simulink model "tempReflexBlockBKP"  (R2016b)
settings: Solver=VariableStepAuto  StartTime=0.0  StopTime=10.0  RelTol=1e-3
settings Model: Creator=Alexander  LastModifiedBy=Alexander

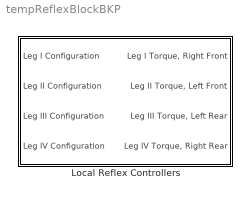
== system tempReflexBlockBKP ==
  "Local Reflex Controllers " : Subsystem

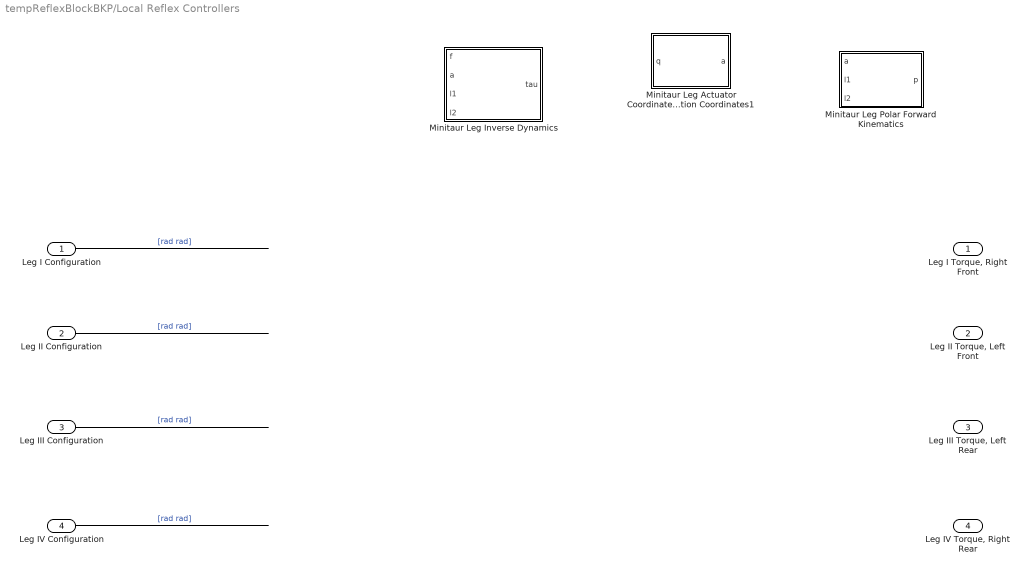
== system tempReflexBlockBKP/Local Reflex Controllers  ==
  Leg I Configuration : Inport  PortDimensions=2
  Leg II Configuration : Inport  Port=2  PortDimensions=2
  Leg III Configuration : Inport  Port=3  PortDimensions=2
  Leg IV Configuration : Inport  Port=4  PortDimensions=2
  Minitaur Leg Actuator Coordinates to Configuration Coordinates1 : MATLAB Function  TreatAsAtomicUnit=on
  Minitaur Leg Inverse Dynamics : MATLAB Function  TreatAsAtomicUnit=on
  Minitaur Leg Polar Forward Kinematics : MATLAB Function  TreatAsAtomicUnit=on
  "Leg I Torque, Right Front" : Outport
  "Leg II Torque, Left Front" : Outport  Port=2
  "Leg III Torque, Left Rear" : Outport  Port=3
  "Leg IV Torque, Right Rear" : Outport  Port=4
  wires:
  Leg I Configuration/1 -> ?  "[rad rad]"
  ? -> "Leg I Torque, Right Front"/1  "[Nm Nm]"
  Leg II Configuration/1 -> ?  "[rad rad]"
  Leg III Configuration/1 -> ?  "[rad rad]"
  Leg IV Configuration/1 -> ?  "[rad rad]"
  ? -> "Leg II Torque, Left Front"/1  "[Nm Nm]"
  ? -> "Leg III Torque, Left Rear"/1  "[Nm Nm]"
  ? -> "Leg IV Torque, Right Rear"/1  "[Nm Nm]"

== matlab function tempReflexBlockBKP/Local Reflex Controllers /Minitaur Leg Actuator Coordinates to Configuration Coordinates1 ==
  data: a output; q input
function a = legActToConfig(q)
% Converts from actuator coordinates q = [theta_A theta_B] to leg
% configuration a = [alpha beta].

    a = [pi 0]' + 0.5*[1 1; 1 -1]*q;

end

== matlab function tempReflexBlockBKP/Local Reflex Controllers /Minitaur Leg Inverse Dynamics ==
  data: f input; tau output; a input; l1 input; l2 input
function tau = legInvDynamics(f,a,l1,l2)
% Computes the actuator torques corresponding to the desired end-effector
% force. Implements tau = J'f, where J is the J' is the leg jacobian
% transpose.

    % Compute leg jacobian
    B = a(2);
    dRdB = l1*sin(B)-(l1^2*sin(B)*cos(B))/sqrt(l2^2-(l1*sin(B))^2);
%     J = 0.5*[1 1; dRdB -1];

    J = 0.5*[1 1; -dRdB 1];
    
    % Compute actuator torques
    tau = J'*f;
    
end

== matlab function tempReflexBlockBKP/Local Reflex Controllers /Minitaur Leg Polar Forward Kinematics ==
  data: a input; p output; l1 input; l2 input
function p = legPolarFK(a,l1,l2)
% Computes the forward kinematics for the minitaur leg in polar
% coordinates.
% a = [alpha beta] are the leg configuration parameters

    p = zeros(2,1);
    p(1) = a(1);
    p(2) = sqrt(l2^2-(l1*sin(a(2)))^2)-l1*cos(a(2));
    
end
